simulink model "Compression_Gain_Calc"  (R2019a)
settings: Solver=FixedStepDiscrete  StartTime=0.0  StopTime=t_end  RelTol=1e-3
InitFcn:
  | clear;
  | DIAGNOSTIC = 0;  %% flag to give more information as simulation proceeds such as comments & plots
  | CALIB_DIAGNOSTIC =  0; %% flag to give more information about calibration of filterbank due to overlap between filters: Mar 2016
  | PRESCRIPT = 1;  %% flag to plot requested versus achieved insertion gains (esp for 125-250 Hz region).
  | ipfiledigrms = -36; %% input file RMS in dB for 65 dB SPL equivalent
  | opfiledigrms = -36; %% output file RMS in dB for 65 dB SPL equivalent
  | equiv_ipSPL = 65; %% simulation of signal at this level through aid`
  | X_high = 1; % Maximum input
  | ref_dB = 85; X_ref = 1; % Define a reference point in X and its dBA value
  | re_level = 10.^(.05*(equiv_ipSPL-65)); %% scale factor at start of hearing aid, to get input to desired simulation level
  | M_bits = 5;   % decides length of tables, 2^(4+M_bits)
  | 
  | NChans = 5;
  | [chan_cfs, chan_thrs, t_atts, t_rels] ...
  |    = InitializeCompressionSettings(NChans);
  | % AidSettings5Chans;
  | 
  | %[VALID_WAV_FILE, sig, Fs, nbits, file_rms_dB, NStreams] ...
  | %  = loadwavfile(ipfiledigrms); %%  find [Fs], performs [recalculate] externally, provided valid file found
  | VALID_WAV_FILE = 1;
  | %[newfile, newpath] = uigetfile('*.wav','Open Signal File To Process.....');
  | %if isequal(newfile,0) || isequal(newpath,0)
  | %    fprintf(1,'\nFile not found'); VALID_WAV_FILE = 0;
  | %else
  | %    [sig, Fs] = audioread(strcat(newpath,newfile));
  | %end
  | X_thresh = 1*10^(0.05*(0-85));
  | 
  | Amplitudes = [X_thresh, X_thresh*10, X_thresh*100, X_thresh*1000, X_thresh*10000, 1]; %, X_thresh*100000];
  | 
  | fMin = 100; %Hz
  | fMax = 10000; %Hz
  | Fs = 48000; %Hz
  | Ts = 1/Fs;
  | %tt = (0:length(sig)-1 )./Fs;
  | tt = 0:Ts:4;
  | deltaF = (fMax - fMin)/tt(end);
  | X_sweep = Amplitudes'*sin(2*pi*(fMin*tt +  0.5*deltaF*tt.*tt)) ;
  | 
  | Fs = 48000;
  | Volume = 6;
  | sig = X_sweep(Volume,:)';
  | opplayer  = audioplayer(sig, Fs);
  | nbits = opplayer.bitspersample;
  | %sig = resample(sig,48000,Fs);
  | %Fs = 48000;
  | 
  | 
  | NStreams = min(size(sig));
  | EQ_SPAN_MSEC = 6;
  | 
  | insrt_frqs = [125, 250, 500, 1000, 2000, 3000, 4000, 6000, 8000, 10000 ]; %% decimal values
  | insrt_gns = [0 3 5 10 15 20 25 30 30 30]; %% prescribed dB for 65 dB input
  | %insrt_gns = 5*ones(1,length(insrt_frqs));  %no prescription
  | n_insrts = length(insrt_gns);
  | 
  | UPPER_FREQ_LIM = min(11e3, 0.90*Fs/2);
  | [ig_eq, calib_bpfs, dig_chan_lvl_0dBgain, dig_chan_dBthrs, Calib_recomb_dBpost] ...
  |     = update_channel_params(Fs, NChans, chan_cfs, chan_thrs, insrt_frqs, insrt_gns, ...
  |     0.1, UPPER_FREQ_LIM, EQ_SPAN_MSEC, PRESCRIPT, DIAGNOSTIC, CALIB_DIAGNOSTIC) ;  %% calculates channel edge frequencies, generates expected band levels for LTASS SWN to calibrate compressors & filterbank
  | ... (+41 lines)
StopFcn:
  | proc_sig = double(out.proc_sig.data(:));
  | %alignedSigs = double(out.alignedSigs.data(:));
  | [opwav, stop_ok] = savewavfile(opfiledigrms, ipfiledigrms, proc_sig, Fs, nbits, NStreams);
  | 
  | load('SweepSimOutput.mat')
  | X_out_Sweep_Sim(Volume,:) = proc_sig;
  | save('SweepSimOutput.mat', 'X_out_Sweep_Sim');
undefined symbols (not defined in the file or in its folder): Ts_system
libraries: simulink x68, hdlsllib x51
(part 2 of 2)

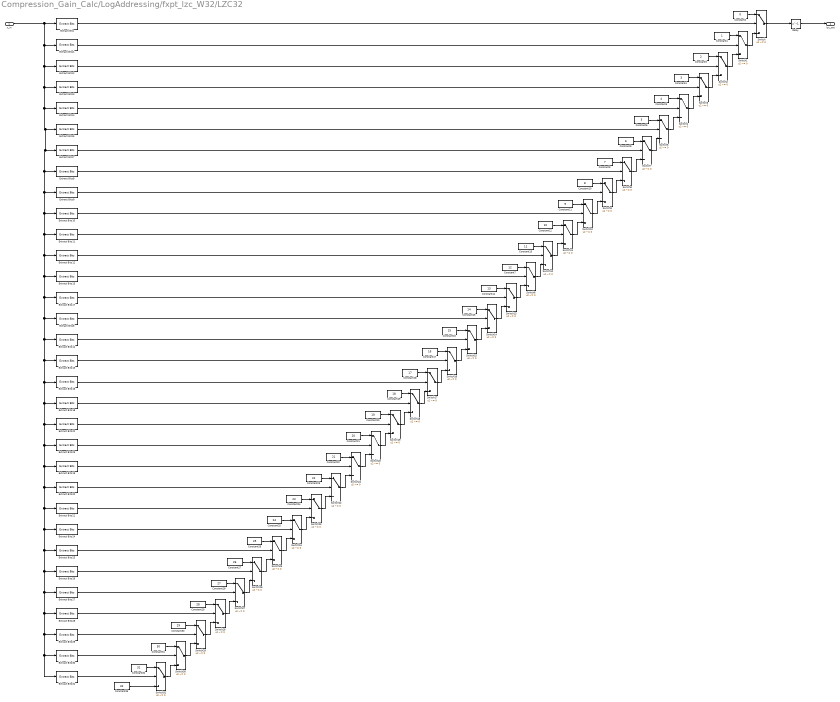
== system Compression_Gain_Calc/LogAddressing/fxpt_lzc_W32/LZC32 ==
  x_in : Inport
  Constant1 : Constant  OutDataTypeStr=fixdt(0,6,0)  SampleTime=Ts_system
  Constant10 : Constant  Value=8  OutDataTypeStr=fixdt(0,6,0)  SampleTime=Ts_system
  Constant11 : Constant  Value=9  OutDataTypeStr=fixdt(0,6,0)  SampleTime=Ts_system
  Constant12 : Constant  Value=10  OutDataTypeStr=fixdt(0,6,0)  SampleTime=Ts_system
  Constant13 : Constant  Value=11  OutDataTypeStr=fixdt(0,6,0)  SampleTime=Ts_system
  Constant14 : Constant  Value=13  OutDataTypeStr=fixdt(0,6,0)  SampleTime=Ts_system
  Constant15 : Constant  Value=14  OutDataTypeStr=fixdt(0,6,0)  SampleTime=Ts_system
  Constant16 : Constant  Value=15  OutDataTypeStr=fixdt(0,6,0)  SampleTime=Ts_system
  Constant17 : Constant  Value=16  OutDataTypeStr=fixdt(0,6,0)  SampleTime=Ts_system
  Constant18 : Constant  Value=17  OutDataTypeStr=fixdt(0,6,0)  SampleTime=Ts_system
  Constant19 : Constant  Value=18  OutDataTypeStr=fixdt(0,6,0)  SampleTime=Ts_system
  Constant2 : Constant  Value=0  OutDataTypeStr=fixdt(0,6,0)  SampleTime=Ts_system
  Constant20 : Constant  Value=19  OutDataTypeStr=fixdt(0,6,0)  SampleTime=Ts_system
  Constant21 : Constant  Value=20  OutDataTypeStr=fixdt(0,6,0)  SampleTime=Ts_system
  Constant22 : Constant  Value=21  OutDataTypeStr=fixdt(0,6,0)  SampleTime=Ts_system
  Constant23 : Constant  Value=22  OutDataTypeStr=fixdt(0,6,0)  SampleTime=Ts_system
  Constant24 : Constant  Value=23  OutDataTypeStr=fixdt(0,6,0)  SampleTime=Ts_system
  Constant25 : Constant  Value=24  OutDataTypeStr=fixdt(0,6,0)  SampleTime=Ts_system
  Constant26 : Constant  Value=25  OutDataTypeStr=fixdt(0,6,0)  SampleTime=Ts_system
  Constant27 : Constant  Value=26  OutDataTypeStr=fixdt(0,6,0)  SampleTime=Ts_system
  Constant28 : Constant  Value=27  OutDataTypeStr=fixdt(0,6,0)  SampleTime=Ts_system
  Constant29 : Constant  Value=28  OutDataTypeStr=fixdt(0,6,0)  SampleTime=Ts_system
  Constant3 : Constant  Value=2  OutDataTypeStr=fixdt(0,6,0)  SampleTime=Ts_system
  Constant30 : Constant  Value=29  OutDataTypeStr=fixdt(0,6,0)  SampleTime=Ts_system
  Constant31 : Constant  Value=30  OutDataTypeStr=fixdt(0,6,0)  SampleTime=Ts_system
  Constant32 : Constant  Value=31  OutDataTypeStr=fixdt(0,6,0)  SampleTime=Ts_system
  Constant33 : Constant  Value=32  OutDataTypeStr=fixdt(0,6,0)  SampleTime=Ts_system
  Constant4 : Constant  Value=3  OutDataTypeStr=fixdt(0,6,0)  SampleTime=Ts_system
  Constant5 : Constant  Value=4  OutDataTypeStr=fixdt(0,6,0)  SampleTime=Ts_system
  Constant6 : Constant  Value=5  OutDataTypeStr=fixdt(0,6,0)  SampleTime=Ts_system
  Constant7 : Constant  Value=12  OutDataTypeStr=fixdt(0,6,0)  SampleTime=Ts_system
  Constant8 : Constant  Value=6  OutDataTypeStr=fixdt(0,6,0)  SampleTime=Ts_system
  Constant9 : Constant  Value=7  OutDataTypeStr=fixdt(0,6,0)  SampleTime=Ts_system
  Delay : Delay  DelayLength=1  InitialCondition=3  SampleTime=Ts_system
  Extract Bits : simulink/Logic and Bit Operations/Extract Bits  bitsToExtract=Range of bits  numBits=8  bitIdxRange=[31 31]  outScalingMode=Treat bit field as an integer
      settings: SourceProductName=Simulink
  Extract Bits1 : simulink/Logic and Bit Operations/Extract Bits  bitsToExtract=Range of bits  numBits=8  bitIdxRange=[30 30]  outScalingMode=Treat bit field as an integer
      settings: SourceProductName=Simulink
  Extract Bits10 : simulink/Logic and Bit Operations/Extract Bits  bitsToExtract=Range of bits  numBits=8  bitIdxRange=[22 22]  outScalingMode=Treat bit field as an integer
      settings: SourceProductName=Simulink
  Extract Bits11 : simulink/Logic and Bit Operations/Extract Bits  bitsToExtract=Range of bits  numBits=8  bitIdxRange=[21 21]  outScalingMode=Treat bit field as an integer
      settings: SourceProductName=Simulink
  Extract Bits12 : simulink/Logic and Bit Operations/Extract Bits  bitsToExtract=Range of bits  numBits=8  bitIdxRange=[20 20]  outScalingMode=Treat bit field as an integer
      settings: SourceProductName=Simulink
  Extract Bits13 : simulink/Logic and Bit Operations/Extract Bits  bitsToExtract=Range of bits  numBits=8  bitIdxRange=[19 19]  outScalingMode=Treat bit field as an integer
      settings: SourceProductName=Simulink
  Extract Bits14 : simulink/Logic and Bit Operations/Extract Bits  bitsToExtract=Range of bits  numBits=8  bitIdxRange=[16 16]  outScalingMode=Treat bit field as an integer
      settings: SourceProductName=Simulink
  Extract Bits15 : simulink/Logic and Bit Operations/Extract Bits  bitsToExtract=Range of bits  numBits=8  bitIdxRange=[15 15]  outScalingMode=Treat bit field as an integer
      settings: SourceProductName=Simulink
  Extract Bits16 : simulink/Logic and Bit Operations/Extract Bits  bitsToExtract=Range of bits  numBits=8  bitIdxRange=[14 14]  outScalingMode=Treat bit field as an integer
      settings: SourceProductName=Simulink
  Extract Bits17 : simulink/Logic and Bit Operations/Extract Bits  bitsToExtract=Range of bits  numBits=8  bitIdxRange=[18 18]  outScalingMode=Treat bit field as an integer
      settings: SourceProductName=Simulink
  Extract Bits18 : simulink/Logic and Bit Operations/Extract Bits  bitsToExtract=Range of bits  numBits=8  bitIdxRange=[13 13]  outScalingMode=Treat bit field as an integer
      settings: SourceProductName=Simulink
  Extract Bits19 : simulink/Logic and Bit Operations/Extract Bits  bitsToExtract=Range of bits  numBits=8  bitIdxRange=[10 10]  outScalingMode=Treat bit field as an integer
      settings: SourceProductName=Simulink
  Extract Bits2 : simulink/Logic and Bit Operations/Extract Bits  bitsToExtract=Range of bits  numBits=8  bitIdxRange=[29 29]  outScalingMode=Treat bit field as an integer
      settings: SourceProductName=Simulink
  Extract Bits20 : simulink/Logic and Bit Operations/Extract Bits  bitsToExtract=Range of bits  numBits=8  bitIdxRange=[9 9]  outScalingMode=Treat bit field as an integer
      settings: SourceProductName=Simulink
  Extract Bits21 : simulink/Logic and Bit Operations/Extract Bits  bitsToExtract=Range of bits  numBits=8  bitIdxRange=[8 8]  outScalingMode=Treat bit field as an integer
      settings: SourceProductName=Simulink
  Extract Bits22 : simulink/Logic and Bit Operations/Extract Bits  bitsToExtract=Range of bits  numBits=8  bitIdxRange=[12 12]  outScalingMode=Treat bit field as an integer
      settings: SourceProductName=Simulink
  Extract Bits23 : simulink/Logic and Bit Operations/Extract Bits  bitsToExtract=Range of bits  numBits=8  bitIdxRange=[11 11]  outScalingMode=Treat bit field as an integer
      settings: SourceProductName=Simulink
  Extract Bits24 : simulink/Logic and Bit Operations/Extract Bits  bitsToExtract=Range of bits  numBits=8  bitIdxRange=[7 7]  outScalingMode=Treat bit field as an integer
      settings: SourceProductName=Simulink
  Extract Bits25 : simulink/Logic and Bit Operations/Extract Bits  bitsToExtract=Range of bits  numBits=8  bitIdxRange=[6 6]  outScalingMode=Treat bit field as an integer
      settings: SourceProductName=Simulink
  Extract Bits26 : simulink/Logic and Bit Operations/Extract Bits  bitsToExtract=Range of bits  numBits=8  bitIdxRange=[5 5]  outScalingMode=Treat bit field as an integer
      settings: SourceProductName=Simulink
  Extract Bits27 : simulink/Logic and Bit Operations/Extract Bits  bitsToExtract=Range of bits  numBits=8  bitIdxRange=[4 4]  outScalingMode=Treat bit field as an integer
      settings: SourceProductName=Simulink
  Extract Bits28 : simulink/Logic and Bit Operations/Extract Bits  bitsToExtract=Range of bits  numBits=8  bitIdxRange=[3 3]  outScalingMode=Treat bit field as an integer
      settings: SourceProductName=Simulink
  Extract Bits29 : simulink/Logic and Bit Operations/Extract Bits  bitsToExtract=Range of bits  numBits=8  bitIdxRange=[2 2]  outScalingMode=Treat bit field as an integer
      settings: SourceProductName=Simulink
  Extract Bits3 : simulink/Logic and Bit Operations/Extract Bits  bitsToExtract=Range of bits  numBits=8  bitIdxRange=[28 28]  outScalingMode=Treat bit field as an integer
      settings: SourceProductName=Simulink
  Extract Bits30 : simulink/Logic and Bit Operations/Extract Bits  bitsToExtract=Range of bits  numBits=8  bitIdxRange=[1 1]  outScalingMode=Treat bit field as an integer
      settings: SourceProductName=Simulink
  Extract Bits31 : simulink/Logic and Bit Operations/Extract Bits  bitsToExtract=Range of bits  numBits=8  bitIdxRange=[0 0]  outScalingMode=Treat bit field as an integer
      settings: SourceProductName=Simulink
  Extract Bits4 : simulink/Logic and Bit Operations/Extract Bits  bitsToExtract=Range of bits  numBits=8  bitIdxRange=[27 27]  outScalingMode=Treat bit field as an integer
      settings: SourceProductName=Simulink
  Extract Bits5 : simulink/Logic and Bit Operations/Extract Bits  bitsToExtract=Range of bits  numBits=8  bitIdxRange=[26 26]  outScalingMode=Treat bit field as an integer
      settings: SourceProductName=Simulink
  Extract Bits6 : simulink/Logic and Bit Operations/Extract Bits  bitsToExtract=Range of bits  numBits=8  bitIdxRange=[17 17]  outScalingMode=Treat bit field as an integer
      settings: SourceProductName=Simulink
  Extract Bits7 : simulink/Logic and Bit Operations/Extract Bits  bitsToExtract=Range of bits  numBits=8  bitIdxRange=[25 25]  outScalingMode=Treat bit field as an integer
      settings: SourceProductName=Simulink
  Extract Bits8 : simulink/Logic and Bit Operations/Extract Bits  bitsToExtract=Range of bits  numBits=8  bitIdxRange=[24 24]  outScalingMode=Treat bit field as an integer
      settings: SourceProductName=Simulink
  Extract Bits9 : simulink/Logic and Bit Operations/Extract Bits  bitsToExtract=Range of bits  numBits=8  bitIdxRange=[23 23]  outScalingMode=Treat bit field as an integer
      settings: SourceProductName=Simulink
  Switch{,1..31} (32 alike) : Switch  Criteria=u2 ~= 0
  lzc_out : Outport
  wires:
  x_in/1 -> Extract Bits31/1, Extract Bits30/1, Extract Bits29/1, Extract Bits28/1, Extract Bits27/1, Extract Bits26/1, Extract Bits25/1, Extract Bits24/1, Extract Bits21/1, Extract Bits20/1, Extract Bits19/1, Extract Bits23/1, Extract Bits22/1, Extract Bits18/1, Extract Bits16/1, Extract Bits15/1, Extract Bits14/1, Extract Bits6/1, Extract Bits17/1, Extract Bits13/1, Extract Bits12/1, Extract Bits11/1, Extract Bits10/1, Extract Bits9/1, Extract Bits8/1, Extract Bits7/1, Extract Bits5/1, Extract Bits4/1, Extract Bits3/1, Extract Bits2/1, Extract Bits1/1, Extract Bits/1
  Switch4/1 -> Switch3/3
  Extract Bits31/1 -> Switch31/2
  Constant28/1 -> Switch27/1
  Switch2/1 -> Switch1/3
  Extract Bits1/1 -> Switch1/2
  Switch6/1 -> Switch12/3
  Switch5/1 -> Switch4/3
  Constant14/1 -> Switch13/1
  Constant31/1 -> Switch30/1
  Extract Bits/1 -> Switch/2
  Constant33/1 -> Switch31/3
  Switch24/1 -> Switch23/3
  Switch14/1 -> Switch13/3
  Extract Bits27/1 -> Switch27/2
  Constant16/1 -> Switch15/1
  Extract Bits4/1 -> Switch4/2
  Constant3/1 -> Switch2/1
  Extract Bits30/1 -> Switch30/2
  Constant1/1 -> Switch1/1
  Extract Bits15/1 -> Switch16/2
  Switch3/1 -> Switch2/3
  Extract Bits19/1 -> Switch21/2
  Extract Bits2/1 -> Switch2/2
  Switch26/1 -> Switch25/3
  Switch18/1 -> Switch17/3
  Extract Bits21/1 -> Switch23/2
  Extract Bits28/1 -> Switch28/2
  Switch29/1 -> Switch28/3
  Switch20/1 -> Switch19/3
  Extract Bits14/1 -> Switch15/2
  Extract Bits23/1 -> Switch20/2
  Constant15/1 -> Switch14/1
  Extract Bits6/1 -> Switch14/2
  Constant17/1 -> Switch16/1
  Extract Bits5/1 -> Switch5/2
  Extract Bits18/1 -> Switch18/2
  Extract Bits20/1 -> Switch22/2
  Extract Bits26/1 -> Switch26/2
  Extract Bits22/1 -> Switch19/2
  Switch11/1 -> Switch10/3
  Extract Bits12/1 -> Switch12/2
  Extract Bits17/1 -> Switch13/2
  Extract Bits24/1 -> Switch24/2
  Switch28/1 -> Switch27/3
  Constant11/1 -> Switch10/1
  Constant8/1 -> Switch7/1
  Extract Bits25/1 -> Switch25/2
  Switch16/1 -> Switch15/3
  Extract Bits29/1 -> Switch29/2
  Switch9/1 -> Switch8/3
  Switch31/1 -> Switch30/3
  Switch19/1 -> Switch18/3
  Extract Bits9/1 -> Switch9/2
  Switch7/1 -> Switch5/3
  Extract Bits13/1 -> Switch6/2
  Extract Bits11/1 -> Switch11/2
  Constant18/1 -> Switch17/1
  Constant4/1 -> Switch3/1
  Extract Bits10/1 -> Switch10/2
  Extract Bits8/1 -> Switch8/2
  Extract Bits7/1 -> Switch7/2
  Constant2/1 -> Switch/1
  Constant22/1 -> Switch21/1
  Switch15/1 -> Switch14/3
  Switch30/1 -> Switch29/3
  Switch13/1 -> Switch6/3
  Switch17/1 -> Switch16/3
  Constant7/1 -> Switch6/1
  Constant30/1 -> Switch29/1
  Constant29/1 -> Switch28/1
  Switch27/1 -> Switch26/3
  Constant32/1 -> Switch31/1
  Constant26/1 -> Switch25/1
  Constant27/1 -> Switch26/1
  Switch25/1 -> Switch24/3
  Constant25/1 -> Switch24/1
  Constant10/1 -> Switch9/1
  Switch12/1 -> Switch11/3
  Switch8/1 -> Switch7/3
  Constant12/1 -> Switch11/1
  Switch21/1 -> Switch20/3
  Switch10/1 -> Switch9/3
  Constant13/1 -> Switch12/1
  Constant9/1 -> Switch8/1
  Constant23/1 -> Switch22/1
  Constant24/1 -> Switch23/1
  Switch22/1 -> Switch21/3
  Switch23/1 -> Switch22/3
  Constant20/1 -> Switch19/1
  Constant21/1 -> Switch20/1
  Constant19/1 -> Switch18/1
  Extract Bits16/1 -> Switch17/2
  Switch1/1 -> Switch/3
  Constant5/1 -> Switch4/1
  Constant6/1 -> Switch5/1
  Extract Bits3/1 -> Switch3/2
  Switch/1 -> Delay/1
  Delay/1 -> lzc_out/1
